simulink model "separator"  (R2017b)
settings: Solver=VariableStepAuto  StartTime=0.0  StopTime=100.0  RelTol=1e-3
settings Model: Creator=Bailey Brookes  LastModifiedBy=Bailey Brookes

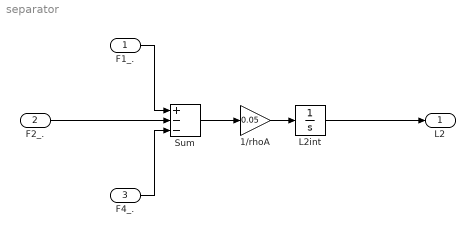
== system separator ==
  F1_. : Inport
  F2_. : Inport  Port=2
  F4_. : Inport  Port=3
  1/rhoA : Gain  Gain=0.05
  L2int : Integrator
  Sum : Sum  Inputs=+--
  L2 : Outport
  wires:
  Sum/1 -> 1/rhoA/1
  F2_./1 -> Sum/2
  L2int/1 -> L2/1
  F1_./1 -> Sum/1
  1/rhoA/1 -> L2int/1
  F4_./1 -> Sum/3
